simulink model "Wah"  (R2020a)
settings: Solver=VariableStepAuto  StartTime=0.0  StopTime=inf  RelTol=1e-3
model workspace (MAT data in the model file):
  Slider = 1
  Variation = 11025
libraries: audiosources x1, dspsnks4 x1, dspfdesign x1, dspsrcs4 x1
settings Model: Creator=Zach Jones  LastModifiedBy=Zach Jones

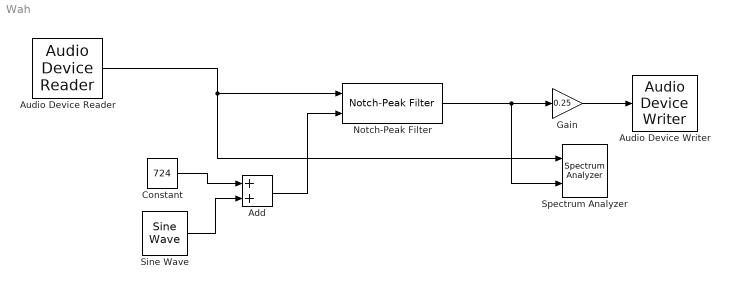
== system Wah ==
  Add : Sum
  Audio Device Reader : audiosources/Audio Device Reader  Driver=DirectSound  Device=Microphone (iMic USB audio system)  SampleRate=44100  NumChannels=1  SamplesPerFrame=1024  BitDepth=16-bit integer  NumBuffers=10  DefaultInputChannelMapping=on  InputChannelMapping=1:2  OutputNumOverrunSamples=off  OutputDataType=double  DriverIdx=1  DeviceWarnFlag=''
      settings: SourceProductBaseCode=AU
  Audio Device Writer : dspsnks4/Audio Device Writer  Driver=DirectSound  Device=Headphones (Realtek(R) Audio)  InheritSampleRate=on  SampleRate=44100  BitDepth=16-bit integer  BufferSize=4096  NumBuffers=10  DefaultOutputChannelMapping=on  OutputChannelMapping=1:2  OutputNumUnderrunSamples=off  DriverIdx=1  DeviceWarnFlag=''
  Constant : Constant  Value=724
  Gain : Gain  Gain=0.25
  Notch-Peak Filter : dspfdesign/Notch-Peak Filter  Specification=Quality factor and center frequency  BandwidthPort=off  Bandwidth=2205  QualityFactorPort=off  QualityFactor=5  CenterFrequencyPort=on  CenterFrequency=1448.339128843338  BandwidthCoefficientPort=off  BandwidthCoefficient=0.72654  CenterFrequencyCoefficientPort=off  CenterFrequencyCoefficient=0.6181818181818182  Output=Peak  InheritSampleRate=off  SampleRate=44100  SimulateUsing=Code generation
      settings: SourceProductBaseCode=DS
  Sine Wave : dspsrcs4/Sine Wave  Amplitude=300  Frequency=1.5  Phase=0  SampleMode=Discrete  OutComplex=Real  CompMethod=Trigonometric fcn  TableSize=Speed  SampleTime=1/44100*1024  SamplesPerFrame=1  ResetState=Restart at time zero  OutputFrames=off  dataType=double  wordLen=16  udDataType=sfix(16)  fracBitsMode=Best precision  numFracBits=15  OutDataTypeStr=double  LastOutDataTypeStr=double
  Spectrum Analyzer : SpectrumAnalyzer  NumInputPorts=2
  wires:
  Audio Device Reader/1 -> Spectrum Analyzer/1, Notch-Peak Filter/1
  Notch-Peak Filter/1 -> Gain/1, Spectrum Analyzer/2
  Constant/1 -> Add/1
  Sine Wave/1 -> Add/2
  Add/1 -> Notch-Peak Filter/2
  Gain/1 -> Audio Device Writer/1
